simulink model "Dynamics_CTC_Matlab"  (R2022a)
settings: Solver=FixedStepAuto  StartTime=0.0  StopTime=30  FixedStep=0.001  RelTol=1e-3
settings Model: Creator=moham  LastModifiedBy=Mohammed Ashraf
settings SolverCC: AlgebraicLoopSolver=TrustRegion
settings DataIOCC: ReturnWorkspaceOutputs=off
settings DebuggingCC: UnconnectedInputMsg=warning  UnconnectedOutputMsg=warning  UnconnectedLineMsg=warning  SFMachineParentedDataDiag=warning  ArithmeticOperatorsInVariantConditions=warning
settings SFSimCC: SimUseLocalCustomCode=off  CustomCodeUndefinedFunction=UseInterfaceOnly
settings RTWCC: RTWUseLocalCustomCode=off

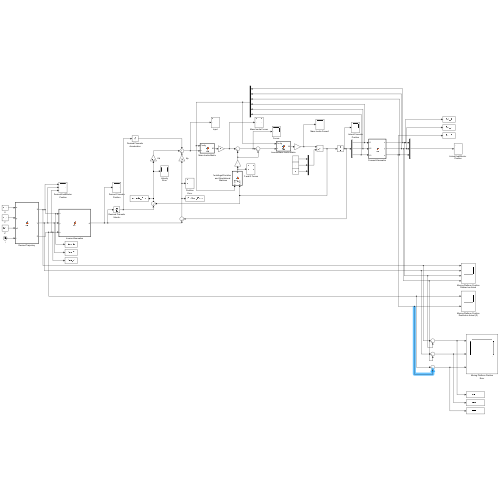
[thumbnail: Simulink's stored preview of the top-level diagram]
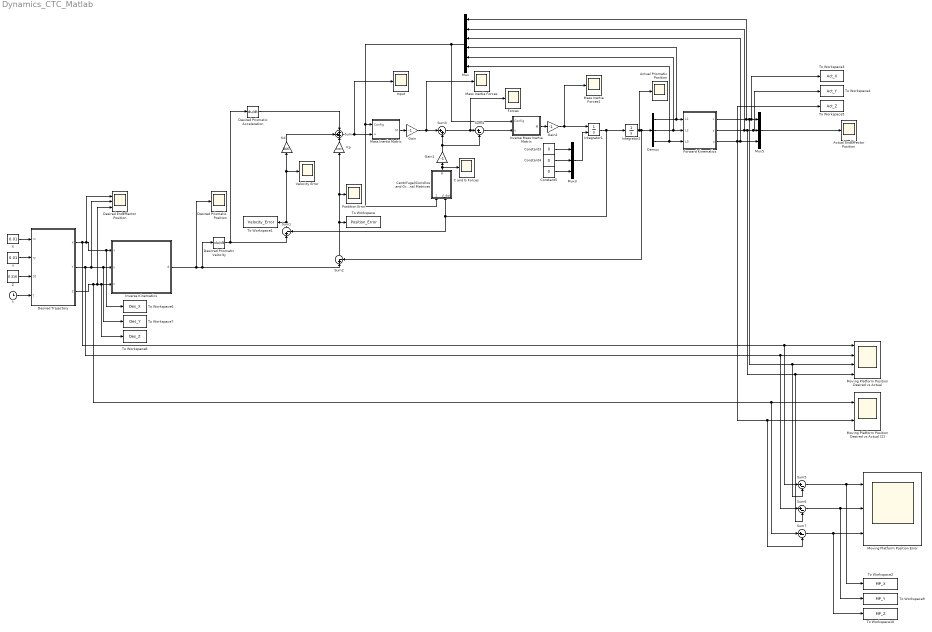
== system Dynamics_CTC_Matlab ==
  Actual EndEffector Position : Scope
  Actual Prismatic Position : Scope
  C and G Forces : Scope
  "Centrifugal/Coriollos and Gravitational Matrices       " : MATLAB Function  TreatAsAtomicUnit=on
  Constant3 : Constant  Value=0
  Constant4 : Constant  Value=0
  Constant5 : Constant  Value=0
  Demux : Demux  Outputs=3
  Desired EndEffector Position : Scope  NumInputPorts=3
  "Desired Prismatic Acceleration " : Derivative
  Desired Prismatic Position : Scope
  Desired Trajectory : MATLAB Function  TreatAsAtomicUnit=on
  Desirred Prismatic Velocity : Derivative
  Forces : Scope
  Forward Kinematics : MATLAB Function  TreatAsAtomicUnit=on
  Gain : Gain  Gain=-1
  Gain1 : Gain  Gain=-1
  Gain2 : Gain  Gain=-1
  Input : Scope
  Integrator1 : Integrator  InitialConditionSource=external
  Integrator2 : Integrator  InitialCondition=0.05  UpperSaturationLimit=0.53  LowerSaturationLimit=0.05
  Inverse Kinematics : MATLAB Function  TreatAsAtomicUnit=on
  Inverse Mass Inertia Matrix : MATLAB Function  TreatAsAtomicUnit=on
  Kd : Gain  Gain=800
  Kp : Gain  Gain=1000
  Mass Inertia Forces : Scope
  Mass Inertia Forces1 : Scope
  Mass Inertia Matrix : MATLAB Function  TreatAsAtomicUnit=on
  Moving Platform Position Desired vs Actual : Scope  NumInputPorts=4
  Moving Platform Position Desired vs Actual (Z) : Scope  NumInputPorts=2
  Moving Platform Position Error : Scope  NumInputPorts=3
  Mux : Mux  Inputs=6
  Mux3 : Mux  Inputs=3
  Mux5 : Mux  Inputs=3
  Postition Error : Scope
  Sum : Sum  Inputs=3
  Sum{1..2,4..7} (6 alike) : Sum  Inputs=|+-
  Sum3 : Sum  Inputs=|++
  To Workspace : ToWorkspace  VariableName=Position_Error  SampleTime=-1
  To Workspace1 : ToWorkspace  VariableName=Velocity_Error  SampleTime=-1
  To Workspace10 : ToWorkspace  VariableName=MP_Z  SampleTime=-1
  To Workspace2 : ToWorkspace  VariableName=MP_X  SampleTime=-1
  To Workspace3 : ToWorkspace  VariableName=Act_X  SampleTime=-1
  To Workspace4 : ToWorkspace  VariableName=Act_Y  SampleTime=-1
  To Workspace5 : ToWorkspace  VariableName=Act_Z  SampleTime=-1
  To Workspace6 : ToWorkspace  VariableName=Des_X  SampleTime=-1
  To Workspace7 : ToWorkspace  VariableName=Des_Y  SampleTime=-1
  To Workspace8 : ToWorkspace  VariableName=Des_Z  SampleTime=-1
  To Workspace9 : ToWorkspace  VariableName=MP_Y  SampleTime=-1
  Velocity Error : Scope
  X : Constant  Value=0.01
  Y : Constant  Value=0.01
  Z : Constant  Value=0.316
  t : Clock
  wires:
  Sum/1 -> Input/1, Mass Inertia Matrix/2(u)
  Kp/1 -> Sum/3
  Mux5/1 -> Actual EndEffector Position/1
  t/1 -> Desired Trajectory/4(t)
  Kd/1 -> Sum/2
  Y/1 -> Desired Trajectory/2(ry)
  Sum2/1 -> To Workspace/1, Postition Error/1, Kp/1
  Mux/1 -> Mass Inertia Matrix/1(Config), "Centrifugal/Coriollos and Gravitational Matrices       "/1(Config), Inverse Mass Inertia Matrix/1(Config)
  Z/1 -> Desired Trajectory/3(z0)
  "Desired Prismatic Acceleration "/1 -> Sum/1
  X/1 -> Desired Trajectory/1(rx)
  Sum4/1 -> Inverse Mass Inertia Matrix/2(u)
  Constant3/1 -> Mux3/1
  Constant4/1 -> Mux3/2
  Constant5/1 -> Mux3/3
  Mux3/1 -> Integrator1/2
  Sum1/1 -> Velocity Error/1, Kd/1, To Workspace1/1
  Demux/1 -> Forward Kinematics/1(L1), Mux/4
  Demux/3 -> Forward Kinematics/3(L3), Mux/6
  Demux/2 -> Forward Kinematics/2(L2), Mux/5
  Inverse Kinematics/1(d) -> Sum2/1, Desirred Prismatic Velocity/1, Desired Prismatic Position/1
  Integrator2/1 -> Sum2/2, Demux/1, Actual Prismatic Position/1
  Desirred Prismatic Velocity/1 -> Sum1/1, "Desired Prismatic Acceleration "/1
  Integrator1/1 -> Integrator2/1, Sum1/2, "Centrifugal/Coriollos and Gravitational Matrices       "/2(d_dot)
  Sum3/1 -> Forces/1, Sum4/1
  Mass Inertia Matrix/1(M) -> Gain/1
  Inverse Mass Inertia Matrix/1(M) -> Gain2/1
  "Centrifugal/Coriollos and Gravitational Matrices       "/1(R) -> Gain1/1, C and G Forces/1
  Gain/1 -> Mass Inertia Forces/1, Sum3/1
  Gain1/1 -> Sum3/2, Sum4/2
  Gain2/1 -> Integrator1/1, Mass Inertia Forces1/1
  Desired Trajectory/3(Z) -> Sum7/1, Moving Platform Position Desired vs Actual (Z)/1, Desired EndEffector Position/3, To Workspace8/1, Inverse Kinematics/3(z)
  Forward Kinematics/2(y) -> Mux/2, Sum6/2, Moving Platform Position Desired vs Actual/4, To Workspace4/1, Mux5/2
  Desired Trajectory/1(X) -> Sum5/1, Moving Platform Position Desired vs Actual/1, Desired EndEffector Position/1, To Workspace6/1, Inverse Kinematics/1(x)
  Forward Kinematics/3(z) -> Sum7/2, Moving Platform Position Desired vs Actual (Z)/2, To Workspace5/1, Mux/3, Mux5/3
  Desired Trajectory/2(Y) -> Sum6/1, Moving Platform Position Desired vs Actual/2, Desired EndEffector Position/2, To Workspace7/1, Inverse Kinematics/2(y)
  Sum6/1 -> To Workspace9/1, Moving Platform Position Error/2
  Forward Kinematics/1(x) -> Mux/1, To Workspace3/1, Mux5/1, Sum5/2, Moving Platform Position Desired vs Actual/3
  Sum7/1 -> To Workspace10/1, Moving Platform Position Error/3
  Sum5/1 -> To Workspace2/1, Moving Platform Position Error/1

== matlab function Dynamics_CTC_Matlab/Mass Inertia Matrix ==
  data: Config input; u input; M output
function M = fcn(Config, u)

%% Dimensions

% Dimensions of the fixed platform in m
SB = 0.485;
WB = 0.140;
UB = 0.280;

% Dimensions of the moving platform in m

sp = 0.09268;
wp = 0.02675;
up = 0.05351;

% Masses of the moving platform, slider and a link in kilograms, respectively 

mp = 9.8783135266E-02;
ms = 1.1195922174;
ml = 0.1044713488;

% Mass Proportion ratio

w = 0.5;

% Leg length in m

L = 0.365;

%% Velocity Analysis (Done)

% Jacobian Matrices Derivation

%Rz1 = [cosd(300), -sind(300), 0; sind(300), cosd(300), 0; 0, 0, 1];
%Rz2 = [cosd(60), -sind(60), 0; sind(60), cosd(60), 0; 0, 0, 1];

d1 = Config(4);
d2 = Config(5);
d3 = Config(6);

u1 = [ 0; 0; -1 ];                                                       % Unit vector for slider 1
u2 = [ 0; 0; -1 ];                                                       % Unit vector for slider 2
u3 = [ 0; 0; -1 ];                                                       % Unit vector for slider 3

a1 = [ -0.5*SB; -WB; 0 ];
a2 = [  0.5*SB; -WB; 0 ];
a3 = [    0   ;  UB; 0 ];

b1 = [  sp/2;  wp;  0 ];                                                % Vector of moving platform joint 1
b2 = [ -sp/2;  wp;  0 ];                                                % Vector of moving platform joint 2
b3 = [   0  ; -up;  0 ];                                                % Vector of moving platform joint 3

c1 = [ 0.03*cosd(60); 0.03*sind(60); 0];
c2 = [-0.03*cosd(60); 0.03*sind(60); 0];
c3 = [       0      ;-0.03;          0];

%c1 = [0; 0.03; 0];
%c2 = [0; 0.03; 0];
%c3 = [0;-0.03; 0];


P = [ Config(1); Config(2); Config(3) - 0.316];

l1 = (1/L)*( P - a1 - b1 - c1 - d1*u1 );                                     % Vector for link set 1
l2 = (1/L)*( P - a2 - b2 - c2 - d2*u2 );                                     % Vector for link set 2
l3 = (1/L)*( P - a3 - b3 - c3 - d3*u3 );                                     % Vector for link set 3

Jd1 = transpose(l1)/(transpose(l1)*u1);                                 % Jacobian Matrix for slider 1
Jd2 = transpose(l2)/(transpose(l2)*u2);                                 % Jacobian Matrix for slider 2
Jd3 = transpose(l3)/(transpose(l3)*u3);                                 % Jacobian Matrix for slider 3
Jd = [Jd1; Jd2; Jd3];

%Equivalent masses of the moving platform and the slider, respectively

Mp = mp + 2*w*ml;
Ms = ms + (1-w)*ml;

% Mass Matrices of the slider and the moving platfrom

Msv = blkdiag(Ms,Ms,Ms);
Mpv = blkdiag(Mp,Mp,Mp);

% Inverse Dynamics of the mechanism

Mm = Msv + transpose(inv(Jd))*Mpv/Jd;

M = Mm*u;

== matlab function Dynamics_CTC_Matlab/Inverse Kinematics ==
  data: x input; d output; y input; z input
function d = fcn(x,y,z)
SB = 0.485; % meters
WB = 0.140; % meters
UB = 0.280; % meters

sp = 0.09268;
wp = 0.02675;
up = 0.05351;

l = 0.365; % meters

a = SB/2 - sp/2;
b = WB - wp;
c = up - UB;

C1 = x^2 + y^2 + z^2 + a^2 + b^2 + 2*a*x + 2*b*y - l^2;
C2 = x^2 + y^2 + z^2 + a^2 + b^2 - 2*a*x + 2*b*y - l^2 ;
C3 = x^2 + y^2 + z^2 + c^2 + 2*c*y - l^2;

L1 = -z - (z^2 - C1)^0.5 - 0.054; % adding 5 cm offset for prismatic joint width
L2 = -z - (z^2 - C2)^0.5 - 0.054; % adding 5 cm offset for prismatic joint width
L3 = -z - (z^2 - C3)^0.5 - 0.054; % adding 5 cm offset for prismatic joint width

d = [L1; L2; L3];

end

== matlab function Dynamics_CTC_Matlab/Desired Trajectory ==
  data: X output; rx input; Y output; ry input; z0 input; t input; Z output
function [X,Y,Z] = fcn(rx, ry, z0, t)

w = 1;
v = 1;


X =  rx*sin((pi/6)*t);
Y =  ry*cos((pi/6)*t);
Z = -(z0 + ((pi/6)*t)/100);

end

== matlab function Dynamics_CTC_Matlab/Centrifugal//Coriollos and Gravitational Matrices        ==
  data: Config input; d_dot input; R output
function R = fcn(Config, d_dot)

%% Dimensions

% Dimensions of the fixed platform in m
SB = 0.485;
WB = 0.140;
UB = 0.280;

% Dimensions of the moving platform in m

sp = 0.09268;
wp = 0.02675;
up = 0.05351;

% Masses of the moving platform, slider and a link in kilograms, respectively 

 mp = 9.8783135266E-02;
 ms = 1.1195922174;
 ml = 0.1044713488;

% Mass Proportion ratio

w = 0.1;

% Leg length in m

L = 0.365;
g = 9.81;

%% Velocity Analysis (Done)

% Jacobian Matrices Derivation

%Rz1 = [cosd(300), -sind(300), 0; sind(300), cosd(300), 0; 0, 0, 1];
%Rz2 = [cosd(60), -sind(60), 0; sind(60), cosd(60), 0; 0, 0, 1];

d1 = Config(4);
d2 = Config(5);
d3 = Config(6);

u1 = [ 0; 0; -1 ];                                                       % Unit vector for slider 1
u2 = [ 0; 0; -1 ];                                                       % Unit vector for slider 2
u3 = [ 0; 0; -1 ];                                                       % Unit vector for slider 3

a1 = [ -0.5*SB; -WB; 0 ];
a2 = [  0.5*SB; -WB; 0 ];
a3 = [    0   ;  UB; 0 ];

b1 = [  sp/2;  wp;  0 ];                                                % Vector of moving platform joint 1
b2 = [ -sp/2;  wp;  0 ];                                                % Vector of moving platform joint 2
b3 = [   0  ; -up;  0 ];                                                % Vector of moving platform joint 3

c1 = [ 0.03*cosd(60); 0.03*sind(60); 0];
c2 = [-0.03*cosd(60); 0.03*sind(60); 0];
c3 = [       0      ;    -0.03;      0];

P = [ Config(1); Config(2); Config(3) - 0.316];

l1 = (1/L)*( P - a1 - b1 - c1 - d1*u1 );                                     % Vector for link set 1
l2 = (1/L)*( P - a2 - b2 - c2 - d2*u2 );                                     % Vector for link set 2
l3 = (1/L)*( P - a3 - b3 - c3 - d3*u3 );                                     % Vector for link set 3

Jd1 = transpose(l1)/(transpose(l1)*u1);                                 % Jacobian Matrix for slider 1
Jd2 = transpose(l2)/(transpose(l2)*u2);                                 % Jacobian Matrix for slider 2
Jd3 = transpose(l3)/(transpose(l3)*u3);                                 % Jacobian Matrix for slider 3
Jd = [Jd1; Jd2; Jd3];

P_dot = Jd\d_dot;

%% Acceleration Analysis (Done)

h = transpose(P_dot);

% Hessian Matrices

H1 = (1/(L*(transpose(l1)*u1))) * (transpose(eye(3) - u1*Jd1)) * (eye(3) - u1*Jd1);
H2 = (1/(L*(transpose(l2)*u2))) * (transpose(eye(3) - u2*Jd2)) * (eye(3) - u2*Jd2);
H3 = (1/(L*(transpose(l3)*u3))) * (transpose(eye(3) - u3*Jd3)) * (eye(3) - u3*Jd3);

% d_ddot = Jd*P_ddot +V*H*Vv

V = blkdiag(h,h,h);
Vv = [inv(Jd); inv(Jd); inv(Jd)];
H = blkdiag(H1, H2, H3);

%Equivalent masses of the moving platform and the slider, respectively

Mp = mp + 6*w*ml;
Ms = ms + (1-w)*ml;
Mpv = blkdiag(Mp,Mp,Mp);

% Inertial and gravity forces
                                                                            
Gp = [0; -Mp*g; 0];                                                            % The gravity forces of the moving platform
Gs = [0; 0; 0];                                                                % The gravity forces of the sliders

C = - transpose(inv(Jd))*Mpv*(Jd\(V*H*Vv));
G = Gs + transpose(inv(Jd))*Gp;

R = C*d_dot + G;
end

== matlab function Dynamics_CTC_Matlab/Inverse Mass Inertia Matrix ==
  data: Config input; u input; M output
function M = fcn(Config, u)

%% Dimensions

% Dimensions of the fixed platform in m
SB = 0.485;
WB = 0.140;
UB = 0.280;

% Dimensions of the moving platform in m

sp = 0.09268;
wp = 0.02675;
up = 0.05351;

% Masses of the moving platform, slider and a link in kilograms, respectively 

mp = 9.8783135266E-02;
ms = 1.1195922174;
ml = 0.1044713488;

% Mass Proportion ratio

w = 0.5;

% Leg length in m

L = 0.365;

%% Velocity Analysis (Done)

% Jacobian Matrices Derivation

%Rz1 = [cosd(300), -sind(300), 0; sind(300), cosd(300), 0; 0, 0, 1];
%Rz2 = [cosd(60), -sind(60), 0; sind(60), cosd(60), 0; 0, 0, 1];

d1 = Config(4);
d2 = Config(5);
d3 = Config(6);

u1 = [ 0; 0; -1 ];                                                       % Unit vector for slider 1
u2 = [ 0; 0; -1 ];                                                       % Unit vector for slider 2
u3 = [ 0; 0; -1 ];                                                       % Unit vector for slider 3

a1 = [ -0.5*SB; -WB; 0 ];
a2 = [  0.5*SB; -WB; 0 ];
a3 = [    0   ;  UB; 0 ];

b1 = [  sp/2;  wp;  0 ];                                                % Vector of moving platform joint 1
b2 = [ -sp/2;  wp;  0 ];                                                % Vector of moving platform joint 2
b3 = [   0  ; -up;  0 ];                                                % Vector of moving platform joint 3

c1 = [ 0.03*cosd(60); 0.03*sind(60); 0];
c2 = [-0.03*cosd(60); 0.03*sind(60); 0];
c3 = [       0      ;-0.03;          0];

%c1 = [0; 0.03; 0];
%c2 = [0; 0.03; 0];
%c3 = [0;-0.03; 0];


P = [ Config(1); Config(2); Config(3) - 0.316];

l1 = (1/L)*( P - a1 - b1 - c1 - d1*u1 );                                     % Vector for link set 1
l2 = (1/L)*( P - a2 - b2 - c2 - d2*u2 );                                     % Vector for link set 2
l3 = (1/L)*( P - a3 - b3 - c3 - d3*u3 );                                     % Vector for link set 3

Jd1 = transpose(l1)/(transpose(l1)*u1);                                 % Jacobian Matrix for slider 1
Jd2 = transpose(l2)/(transpose(l2)*u2);                                 % Jacobian Matrix for slider 2
Jd3 = transpose(l3)/(transpose(l3)*u3);                                 % Jacobian Matrix for slider 3
Jd = [Jd1; Jd2; Jd3];

%Equivalent masses of the moving platform and the slider, respectively

Mp = mp + 2*w*ml;
Ms = ms + (1-w)*ml;

% Mass Matrices of the slider and the moving platfrom

Msv = blkdiag(Ms,Ms,Ms);
Mpv = blkdiag(Mp,Mp,Mp);

% Inverse Dynamics of the mechanism

Mm = Msv + transpose(inv(Jd))*Mpv/Jd;

M = Mm\u;

== matlab function Dynamics_CTC_Matlab/Forward Kinematics ==
  data: L1 input; x output; L2 input; L3 input; y output; z output
function [x,y,z] = fcn(L1, L2, L3)
SB = 0.485; % meters
WB = 0.140; % meters
UB = 0.280; % meters

sp = 0.09268; % meters
wp = 0.02675; % meters
up = 0.05351; % meters

l = 0.365; % meters

L1 = L1 + 0.054;
L2 = L2 + 0.054;
L3 = L3 + 0.054;

a = SB/2 - sp/2;
b = WB - wp;
c = up - UB;

d = (L2-L1)/(2*a);
e = (L2^2 - L1^2)/(4*a);

D = (L3 - L1 - a*d)/(b-c);
E = (c^2 - a^2 - b^2 - 2*a*e + L3^2 - L1^2)/(2*(b-c));

A = d^2 + D^2 + 1;
B = 2*(d*e + D*E + c*D + L3);
C = e^2 + E^2 + c^2 + 2*c*E + L3^2 - l^2;

z = (-B - (B^2 - 4*A*C)^0.5)/(2*A);
x = d * z + e;
y = D * z + E;
end
